simulink model "GRPsim"  (R2024b)
settings: Solver=VariableStepAuto  StartTime=0.0  StopTime=10.0  RelTol=1e-3
undefined symbols (not defined in the file or in its folder): factstruct
libraries: shared6dof x1, aerolibadyn x1, slpidlib x1
settings Model: Creator=ryanmarquardt  LastModifiedBy=ryanmarquardt

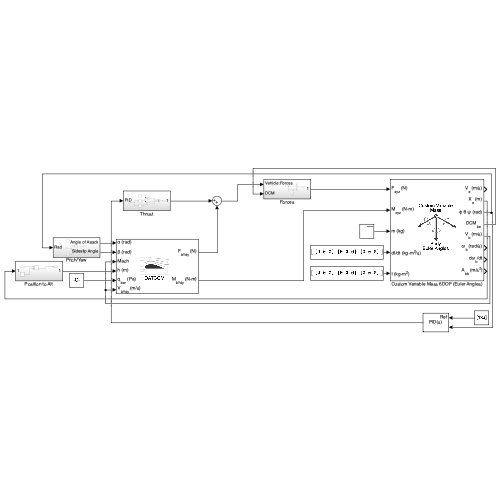
[thumbnail: Simulink's stored preview of the top-level diagram]
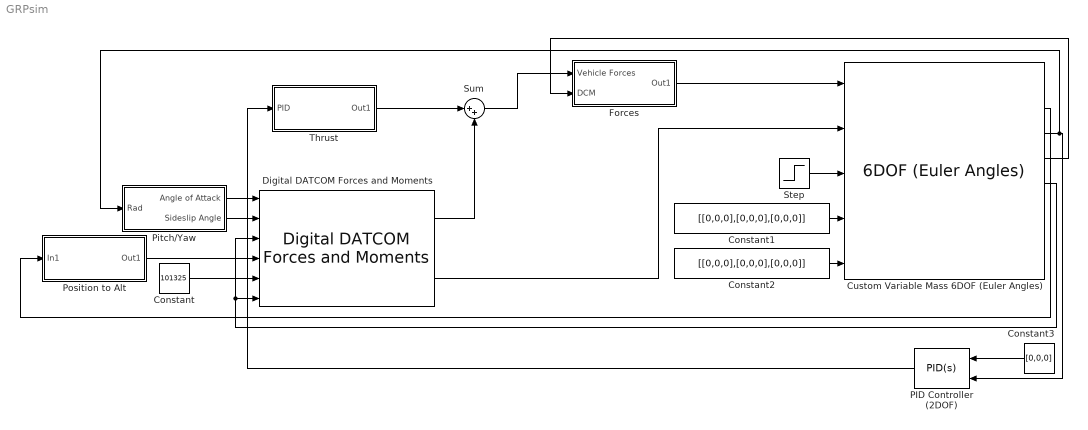
== system GRPsim ==
  Constant : Constant  Value=101325
  Constant1 : Constant  Value=[[0,0,0],[0,0,0],[0,0,0]]
  Constant2 : Constant  Value=[[0,0,0],[0,0,0],[0,0,0]]
  Constant3 : Constant  Value=[0,0,0]
  Custom Variable Mass 6DOF (Euler Angles) : shared6dof/6DOF (Euler Angles)  units=Metric (MKS)  mtype=Custom Variable  rep=Euler Angles  xme_0=[0 0 0]  Vm_0=[0 0 0]  eul_0=[0 0 0]  pm_0=[0 0 0]  mass_0=1.0  mass_e=0.5  mass_f=2.0  inertia=eye(3)  inertia_e=eye(3)  inertia_f=2*eye(3)  k_quat=1.0  vre_flag=off  abi_flag=off  aMode=0  xme_statename=''  Vm_statename=''  eul_statename=''  quat_statename=''  pm_statename=''  mass_statename=''
      settings: LibrarySourceBlock=aerolib6dof2/Custom Variable Mass 6DOF (Euler Angles)
  Digital DATCOM Forces and Moments : aerolibadyn/Digital DATCOM Forces and Moments  units=Metric (MKS)  dcase=factstruct{1}  fmode=Body  buildno=0  imethod=None - flat  emethod=None - clip  rmethod=Clip to Range  action=None
  Forces : Subsystem
  PID Controller (2DOF) : slpidlib/PID Controller (2DOF)  Controller=PID  Form=Parallel  TimeDomain=Continuous-time  UseExternalTs=off  SampleTime=-1  IntegratorMethod=Forward Euler  FilterMethod=Forward Euler  ControllerParametersSource=internal  P=1  I=1  UseKiTs=off  D=0  UseExternalDerivativeSource=off  N=100  UseFilter=on  b=1  c=1  TunerSelectOption=Transfer Function Based (PID Tuner App)  InitialConditionSource=internal  InitialConditionForIntegrator=0  InitialConditionForFilter=0  DifferentiatorICPrevScaledInput=0  ExternalReset=none  TrackingMode=off  Kt=1  LimitOutput=off  SatLimitsSource=internal  UpperSaturationLimit=inf  LowerSaturationLimit=-inf  LinearizeAsGain=on  AntiWindupMode=none  Kb=1  LimitIntegrator=off  UpperIntegratorSaturationLimit=inf  LowerIntegratorSaturationLimit=-inf  POutMin=[]  POutMax=[]  IOutMin=[]  IOutMax=[]  DOutMin=[]  DOutMax=[]  NOutMin=[]  NOutMax=[]  bOutMin=[]  bOutMax=[]  cOutMin=[]  cOutMax=[]  SumOutMin=[]  SumOutMax=[]  SaturationOutMin=[]  SaturationOutMax=[]  PParamMin=[]  PParamMax=[]  IParamMin=[]  IParamMax=[]  DParamMin=[]  DParamMax=[]  NParamMin=[]  NParamMax=[]  bParamMin=[]  bParamMax=[]  cParamMin=[]  cParamMax=[]  KbParamMin=[]  KbParamMax=[]  KtParamMin=[]  KtParamMax=[]  KbOutMin=[]  KbOutMax=[]  KtOutMin=[]  KtOutMax=[]  IntegratorOutMin=[]  IntegratorOutMax=[]  FilterOutMin=[]  FilterOutMax=[]  SumI1OutMin=[]  SumI1OutMax=[]  SumI2OutMin=[]  SumI2OutMax=[]  SumI3OutMin=[]  SumI3OutMax=[]  SumI4OutMin=[]  SumI4OutMax=[]  SumDOutMin=[]  SumDOutMax=[]  Sum1OutMin=[]  Sum1OutMax=[]  Sum2OutMin=[]  Sum2OutMax=[]  Sum3OutMin=[]  Sum3OutMax=[]  DifferentiatorOutMin=[]  DifferentiatorOutMax=[]  FilterDiffOutCoefMin=[]  FilterDiffOutCoefMax=[]  ReciprocalOutMin=[]  ReciprocalOutMax=[]  SumDenOutMin=[]  SumDenOutMax=[]  SumNumOutMin=[]  SumNumOutMax=[]  DivideOutMin=[]  DivideOutMax=[]  UdiffTsProdOutMin=[]  UdiffTsProdOutMax=[]  NTsProdOutMin=[]  NTsProdOutMax=[]  UintegralTsProdOutMin=[]  UintegralTsProdOutMax=[]  UngainTsProdOutMin=[]  UngainTsProdOutMax=[]  ClampingZeroOutDataTypeStr=Inherit: Inherit via back propagation  ClampingZeroOutMin=[]  ClampingZeroOutMax=[]  FilterDenConstantOutDataTypeStr=Inherit: Inherit via back propagation  FilterDenConstantOutMin=[]  FilterDenConstantOutMax=[]  PCopyOutDataTypeStr=Inherit: Inherit via back propagation  PCopyOutMin=[]  PCopyOutMax=[]  NCopyOutDataTypeStr=Inherit: Inherit via back propagation  NCopyOutMin=[]  NCopyOutMax=[]  IntegratorContinuousStateAttributes=''  IntegratorStateMustResolveToSignalObject=off  IntegratorRTWStateStorageClass=Auto  FilterContinuousStateAttributes=''  FilterStateMustResolveToSignalObject=off  FilterRTWStateStorageClass=Auto  ParallelPVariant=InternalParameters  IdealPVariant=Disabled  IVariant=InternalParameters  DVariant=InternalParameters  bVariant=InternalParameters  cVariant=InternalParameters  IntegratorVariant=Continuous  SatVariant=Disabled  AWVariant=Passthrough  PCopyVariant=Disabled  TRVariant=Disabled  FdbkBlocksVariant=Forward  IdealPFdbkVariant=Disabled  SatFdbkVariant=Disabled  DerivativeFilterVariant=ContFilter  NVariant=InternalParameters  NCopyVariant=Disabled  FilterICVariant=InternalICsFilter  IntegratorICVariant=InternalICs  ExternalResetVariant=Disabled  TRSumVariant=Passthrough  SumFdbkVariant=Disabled  SumVariant=Sum_PID  TsampFilterVariant=InternalTs  TsampNgainVariant=Passthrough  TsampIntegralVariant=Passthrough  ExternalSaturationOutDataTypeStr=Inherit: Same as second input  DerivativeSourceVariant=ErrorSignal  PreIntVariant=InternalPreInt
  Pitch/Yaw : Subsystem
  Position to Alt : Subsystem
  Step : Step  SampleTime=0
  Sum : Sum  Inputs=|++
  Thrust : Subsystem
  wires:
  Forces/1(Out1) -> Custom Variable Mass 6DOF (Euler Angles)/1
  Custom Variable Mass 6DOF (Euler Angles)/4 -> Forces/2(DCM)
  Sum/1 -> Forces/1(Vehicle Forces)
  Thrust/1(Out1) -> Sum/1
  Digital DATCOM Forces and Moments/1 -> Sum/2
  Custom Variable Mass 6DOF (Euler Angles)/5 -> Digital DATCOM Forces and Moments/3, Digital DATCOM Forces and Moments/6
  Constant/1 -> Digital DATCOM Forces and Moments/5
  Position to Alt/1(Out1) -> Digital DATCOM Forces and Moments/4
  Digital DATCOM Forces and Moments/2 -> Custom Variable Mass 6DOF (Euler Angles)/2
  PID Controller (2DOF)/1 -> Thrust/1(PID)
  Step/1 -> Custom Variable Mass 6DOF (Euler Angles)/3
  Constant2/1 -> Custom Variable Mass 6DOF (Euler Angles)/5
  Constant1/1 -> Custom Variable Mass 6DOF (Euler Angles)/4
  Custom Variable Mass 6DOF (Euler Angles)/2 -> Position to Alt/1(In1)
  Pitch/Yaw/1(Angle of Attack) -> Digital DATCOM Forces and Moments/1
  Pitch/Yaw/2(Sideslip Angle) -> Digital DATCOM Forces and Moments/2
  Custom Variable Mass 6DOF (Euler Angles)/3 -> PID Controller (2DOF)/2, Pitch/Yaw/1(Rad)
  Constant3/1 -> PID Controller (2DOF)/1

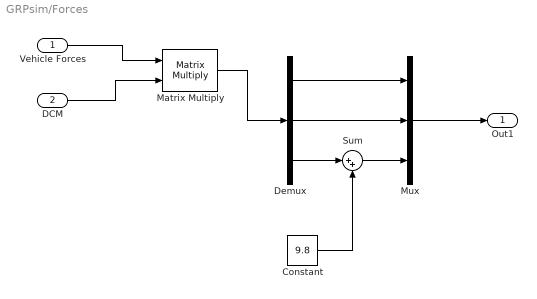
== system GRPsim/Forces ==
  Vehicle Forces : Inport
  DCM : Inport  Port=2
  Constant : Constant  Value=9.8
  Demux : Demux  Outputs=3
  Matrix Multiply : Product  Multiplication=Matrix(*)
  Mux : Mux  Inputs=3
  Sum : Sum  Inputs=|++
  Out1 : Outport
  wires:
  Vehicle Forces/1 -> Matrix Multiply/1
  DCM/1 -> Matrix Multiply/2
  Matrix Multiply/1 -> Demux/1
  Mux/1 -> Out1/1
  Constant/1 -> Sum/2
  Demux/3 -> Sum/1
  Demux/2 -> Mux/2
  Demux/1 -> Mux/1
  Sum/1 -> Mux/3

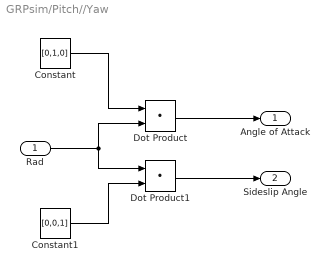
== system GRPsim/Pitch//Yaw ==
  Rad : Inport
  Constant : Constant  Value=[0,1,0]
  Constant1 : Constant  Value=[0,0,1]
  Dot Product : DotProduct  OutDataTypeStr=Inherit: Inherit via internal rule
  Dot Product1 : DotProduct  OutDataTypeStr=Inherit: Inherit via internal rule
  Angle of Attack : Outport
  Sideslip Angle : Outport  Port=2
  wires:
  Constant1/1 -> Dot Product1/2
  Constant/1 -> Dot Product/1
  Rad/1 -> Dot Product/2, Dot Product1/1
  Dot Product/1 -> Angle of Attack/1
  Dot Product1/1 -> Sideslip Angle/1

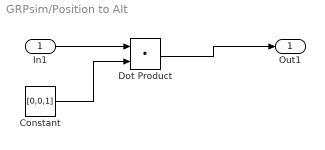
== system GRPsim/Position to Alt ==
  In1 : Inport
  Constant : Constant  Value=[0,0,1]
  Dot Product : DotProduct  OutDataTypeStr=Inherit: Inherit via internal rule
  Out1 : Outport
  wires:
  In1/1 -> Dot Product/1
  Constant/1 -> Dot Product/2
  Dot Product/1 -> Out1/1

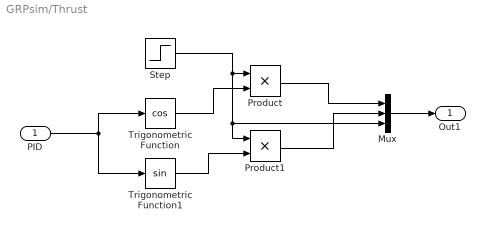
== system GRPsim/Thrust ==
  PID : Inport
  Mux : Mux  Inputs=3
  Product : Product
  Product1 : Product
  Step : Step  SampleTime=0
  Trigonometric Function : Trigonometry  Operator=cos
  Trigonometric Function1 : Trigonometry
  Out1 : Outport
  wires:
  PID/1 -> Trigonometric Function1/1, Trigonometric Function/1
  Trigonometric Function1/1 -> Product1/2
  Trigonometric Function/1 -> Product/2
  Step/1 -> Mux/3, Product1/1, Product/1
  Product/1 -> Mux/1
  Product1/1 -> Mux/2
  Mux/1 -> Out1/1
